simulink model "EV3_MatSys_Demo_USB"  (R2023a)
settings: Solver=FixedStepAuto  StartTime=0.0  StopTime=10.0  FixedStep=0.1  RelTol=1e-3
libraries: realtime_pacer_lib x1
settings Model: Creator=chris  LastModifiedBy=chris

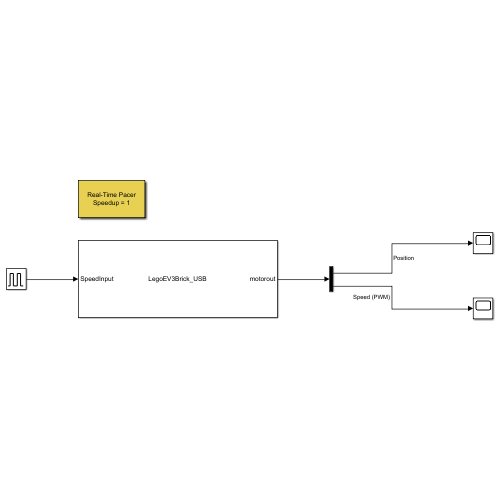
[thumbnail: Simulink's stored preview of the top-level diagram]
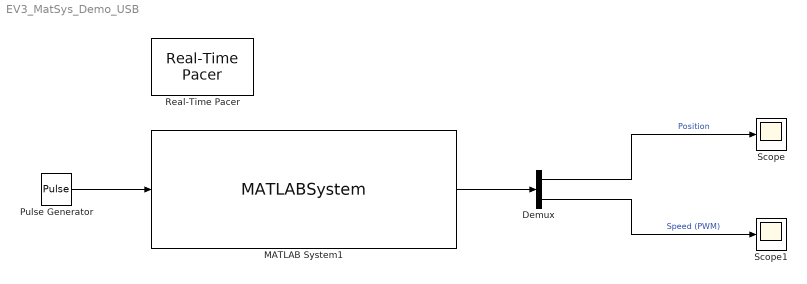
== system EV3_MatSys_Demo_USB ==
  Demux : Demux  Outputs=2
  MATLAB System1 : MATLABSystem  System=LegoEV3Brick_USB  motorport=A  SimulateUsing=Interpreted execution
      mask Type: LegoEV3Brick_USB
      mask Display:
      | disp('LegoEV3Brick_USB');
      | port_label('input',1,'SpeedInput');
      | port_label('output',1,'motorout');
  Pulse Generator : DiscretePulseGenerator  PulseType=Time based  Amplitude=100  Period=5  PulseWidth=50
  Real-Time Pacer : realtime_pacer_lib/Real-Time Pacer  simTimePerRealTime=1
  Scope : Scope
  Scope1 : Scope
  wires:
  Pulse Generator/1 -> MATLAB System1/1
  MATLAB System1/1 -> Demux/1
  Demux/1 -> Scope/1  "Position"
  Demux/2 -> Scope1/1  "Speed (PWM)"
